simulink model "Can_send_receive"  (R2024a)
settings: Solver=FixedStepAuto  StartTime=0.0  StopTime=20  RelTol=1e-3  EnableMultiTasking=on
undefined symbols (not defined in the file): CAN, FD
libraries: stmutilitieslib x31, simulink x22, stm32blockslib x10, canfdmsglib x6, stm32h7xxblockslib x2
settings Model: STM32="{\"FDCANWrite\":[{\"ID\":\"Can_send_receive:103\"},{\"ID\":\"Can_send_receive:112\"},{\"ID\":\"Can_send_receive:559\"},{\"ID\":\"Can_send_receive:574\"},{\"ID\":\"Can_send_receive:617\"},{\"ID\":\"Can_send_receive:630\"},{\"ID\":\"Can_send_receive:677\"},{\"ID\":\"Can_send_receive:678\"}],\"HardwareInterrupt\":[{\"ID\":\"Can_send_receive:135\"},{\"ID\":\"Can_send_receive:278\"}],\"FDCANRead\":[{\"ID\":\"Can_send_receive:127\"},{\"ID\":\"Can_send_receive:282\"}]}"  Creator=ezeki  LastModifiedBy=ezeki
settings SolverCC: PositivePriorityOrder=on  AutoInsertRateTranBlk=on
settings OptimizationCC: DefaultParameterBehavior=Inlined  EnhancedBackFolding=on  PassReuseOutputArgsAs=Individual arguments  ZeroExternalMemoryAtStartup=off  ZeroInternalMemoryAtStartup=off  MaxStackSize=512  OptimizeBlockOrder=speed  DifferentSizesBufferReuse=on  OptimizationCustomize=off  EfficientTunableParamExpr=on
settings DebuggingCC: ParameterTunabilityLossMsg=error
settings HardwareCC: ProdBitPerPointer=32  ProdBitPerSizeT=32  ProdBitPerPtrDiffT=32  ProdLargestAtomicInteger=Long  ProdLargestAtomicFloat=Double  ProdWordSize=32  ProdLongLongMode=on  ProdHWDeviceType=ARM Compatible->ARM Cortex-M
settings SFSimCC: MATLABDynamicMemAlloc=off
settings RTWCC: Description=Embedded Coder  SystemTargetFile=ert.tlc  HardwareBoard=STM32H7xx Based (Single-core)  TLCOptions="-aInlineSetEventsForThisBaseRateFcn=TLC_FALSE -aSuppressMultiTaskScheduler=TLC_FALSE  -aRateBasedStepFcn=0"  TemplateMakefile=ert_default_tmf  Toolchain=GNU Tools for ARM Embedded Processors  BuildConfiguration=Faster Runs
settings CodeAppCC: ForceParamTrailComments=on  IgnoreCustomStorageClasses=off  OperatorAnnotations=on  SimulinkDataObjDesc=on  SFDataObjDesc=on  InsertBlockDesc=on
settings ERTTargetCC: TargetLangStandard=C99 (ISO)  CodeReplacementLibrary=ARM Cortex-M  ExtModeTransport=3  ExtModeStaticAlloc=on  ExtModeStaticAllocSize=2048  ExtModeMexFile=ext_xcp  ExtModeIntrfLevel=Level2 - Open

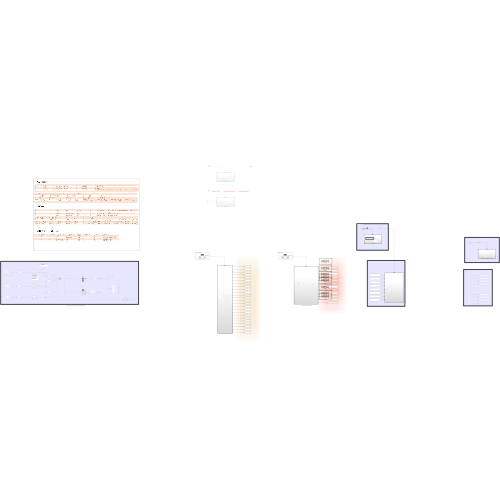
[thumbnail: Simulink's stored preview of the top-level diagram]
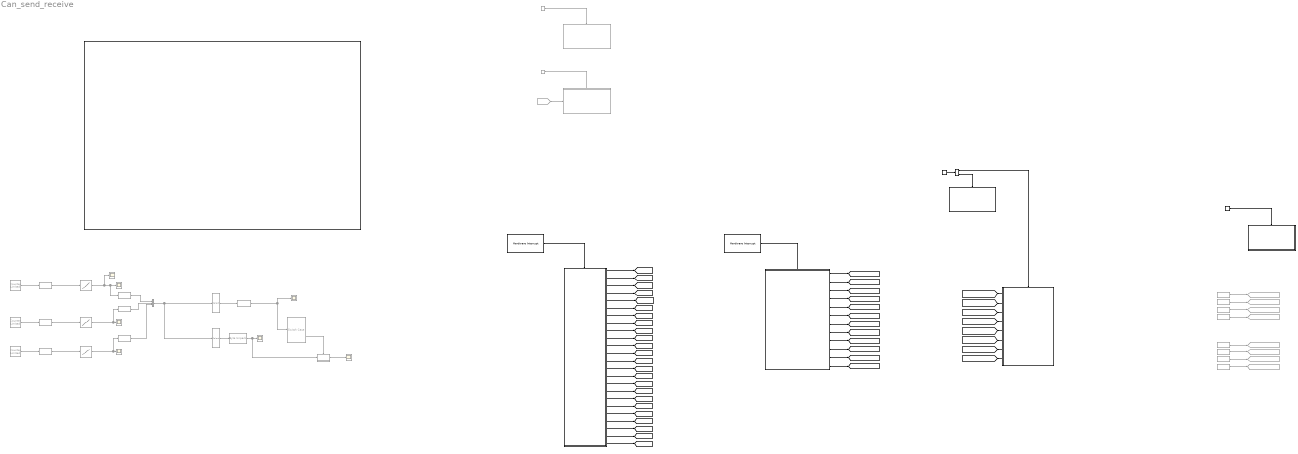
== system Can_send_receive ==
  note: For testing purposes only
  note: CAN 1 information from pedal box and dash.
  note: CAN 2 Receive Data From Inverters
  note: Forwarding Messages From the Inverters to Data Logger
  note: Example On How to send Messages to Inverters
  note: This was made for testing the unmultiplexing of Inverter Messages
  note: Inverter Can Setup
  note: A look up table of CAN ID's which are used to request cyclic transmission of data from the inverters
  note: Counter Selects which ID to send
  note: Byte 0 tells the inverters you are setting up cyclic messaging.
  1-D Lookup Table : Lookup_n-D  Commented=on  NumberOfTableDimensions=1  BreakpointsForDimension1=[0 1 2 3 4 5]  Table=[235 74 168 73 95 138]  InterpMethod=Nearest  InternalRulePriority=Speed  RndMeth=Simplest
  1-D Lookup Table1 : Lookup_n-D  Commented=on  NumberOfTableDimensions=1  BreakpointsForDimension1=[0 1 2 3 4 5]  Table=[25 200 25 200 50 50]  InterpMethod=Nearest  InternalRulePriority=Speed  RndMeth=Simplest
  1-D Lookup Table2 : Lookup_n-D  Commented=on  NumberOfTableDimensions=1  BreakpointsForDimension1=[0 1 2 3 4 5]  Table=[25 200 25 200 50 50]  InterpMethod=Nearest  InternalRulePriority=Speed  RndMeth=Simplest
  10 HZ Send : Subsystem  Commented=on  TreatAsAtomicUnit=on
  10 HZ Send1 : Subsystem  TreatAsAtomicUnit=on
  50 HZ Send Torque Requests to Inverters : Subsystem  TreatAsAtomicUnit=on
  50 HZ Send1 : Subsystem  Commented=on  TreatAsAtomicUnit=on
  Byte Unpack : stmutilitieslib/Byte Unpack  Commented=on  dimensions={[1]}  datatypes={'uint16'}  byteAlign=1  blockPlatform=stm32f4discovery
  Constant{,1..3,5..6,10..11} (8 alike) : Constant  Commented=on  Value=25000
  Counter Limited : simulink/Sources/Counter Limited  Commented=on  uplimit=5  tsamp=0.1
  Counter Limited1 : simulink/Sources/Counter Limited  Commented=on  uplimit=5  tsamp=0.4
  Counter Limited2 : simulink/Sources/Counter Limited  Commented=on  uplimit=5  tsamp=0.7
  Data Type Conversion{1,3,5,16} (4 alike) : DataTypeConversion  Commented=on  OutDataTypeStr=double  SaturateOnIntegerOverflow=off  RndMeth=Floor
  Data Type Conversion2 : DataTypeConversion  Commented=on  OutDataTypeStr=uint8  SaturateOnIntegerOverflow=off  RndMeth=Floor
  Data Type Conversion4 : DataTypeConversion  Commented=on  OutDataTypeStr=uint8  SaturateOnIntegerOverflow=off  RndMeth=Floor
  Data Type Conversion6 : DataTypeConversion  Commented=on  OutDataTypeStr=uint8  SaturateOnIntegerOverflow=off  RndMeth=Floor
  From : From  Commented=on  GotoTag=WSFR
  Function-Call Generator : simulink/Ports & Subsystems/Function-Call Generator  Commented=on  sample_time=0.1  numberOfIterations=1  DisallowWideOutput=off
  Function-Call Generator1 : simulink/Ports & Subsystems/Function-Call Generator  Commented=on  sample_time=0.02  numberOfIterations=1  DisallowWideOutput=off
  Function-Call Generator2 : simulink/Ports & Subsystems/Function-Call Generator  sample_time=0.02  numberOfIterations=1  DisallowWideOutput=off
  Function-Call Generator4 : simulink/Ports & Subsystems/Function-Call Generator  sample_time=0.2  numberOfIterations=1  DisallowWideOutput=off
  Function-Call Split : FunctionCallSplit  IconShape=distinctive  NumOutputPorts=2  OutputPortLayout=default
  Function-Call Subsystem : Subsystem  TreatAsAtomicUnit=on
  Function-Call Subsystem1 : Subsystem  TreatAsAtomicUnit=on
  Goto36 : Goto  Commented=on  GotoTag=CAN_LEFT_Inverter_Bus_Voltage
  Goto37 : Goto  Commented=on  GotoTag=CAN_LEFT_Inverter_Motor_Current
  Goto38 : Goto  Commented=on  GotoTag=CAN_LEFT_Inverter_Motor_Speed
  Goto39 : Goto  Commented=on  GotoTag=CAN_RIGHT_Inverter_Motor_Speed
  Goto41 : Goto  Commented=on  GotoTag=CAN_LEFT_Inverter_Motor_Voltage
  Goto42 : Goto  Commented=on  GotoTag=CAN_RIGHT_Inverter_Bus_Voltage
  Goto45 : Goto  Commented=on  GotoTag=CAN_RIGHT_Inverter_Motor_Current
  Goto47 : Goto  Commented=on  GotoTag=CAN_RIGHT_Inverter_Motor_Voltage
  Hardware Interrupt1 : stm32h7xxblockslib/Hardware Interrupt  ISRGroup=Controller Area Network Flexible Data-Rate (FDCAN)  ISRName=FDCAN2_IT0_IRQHandler  ISRNumber=35  EventsList={ 'off', 'FDCAN2 HPME', '1'; 'off', 'FDCAN2 DRXE', '2'; 'on', 'FDCAN2 RF0NE', '3'; 'off', 'FDCAN2 RF0F', '4'; 'off', 'FDCAN2 RF0L', '5'; 'off', 'FDCAN2 RF0W', '6'; 'off', 'FDCAN2 RF1NE', '7'; 'off', 'FDCAN2 RF1F', '8'; 'off', 'FDCAN2 RF1L', '9'; 'off', 'FDCAN2 RF1W', '10'; 'off', 'FDCAN2 TC', '11'; 'off', 'FDCAN2 TCF', '12'; 'off', 'FDCAN2 TFE', '13'; 'off', 'FDCAN2 TEFN', '14'; 'off', 'FDCAN2 TEFL', '15'; 'off', 'FDCAN2 TEFF', '16'; 'off', 'FDCAN2 TEFW', '17'; 'off', 'FDCAN2 TSW', '18'; 'off', 'FDCAN2 MRAF', '19'; 'off', 'FDCAN2 TOO', '20'; 'off', 'FDCAN2 ELO', '21'; 'off', 'FDCAN2 EP', '22'; 'off', 'FDCAN2 EW', '23'; 'off', 'FDCAN2 BO', '24'; 'off', 'FDCAN2 WDI', '25'; 'off', 'FDCAN2 PEA', '26'; 'off', 'FDCAN2 PED', '27'; 'off', 'FDCAN2 ARA', '28'; 'off', 'Custom event', '29' }  SelectedEvents={'FDCAN2 RF0NE'}  TaskPriority=29  DisablePreemption=off  ClearInterruptFlagsAtEndOfEvent=off  InterruptDefinitionFile=$(TARGET_ROOT)/registry/interrupts/STM32F4xxBased_interrupts.xml  HardwareBoard=STM32H7xx Based  EnableSimPort=off
  Hardware Interrupt3 : stm32h7xxblockslib/Hardware Interrupt  ISRGroup=Controller Area Network Flexible Data-Rate (FDCAN)  ISRName=FDCAN1_IT0_IRQHandler  ISRNumber=34  EventsList={ 'off', 'FDCAN1 HPME', '1'; 'off', 'FDCAN1 DRXE', '2'; 'on', 'FDCAN1 RF0NE', '3'; 'off', 'FDCAN1 RF0F', '4'; 'off', 'FDCAN1 RF0L', '5'; 'off', 'FDCAN1 RF0W', '6'; 'off', 'FDCAN1 RF1NE', '7'; 'off', 'FDCAN1 RF1F', '8'; 'off', 'FDCAN1 RF1L', '9'; 'off', 'FDCAN1 RF1W', '10'; 'off', 'FDCAN1 TC', '11'; 'off', 'FDCAN1 TCF', '12'; 'off', 'FDCAN1 TFE', '13'; 'off', 'FDCAN1 TEFN', '14'; 'off', 'FDCAN1 TEFL', '15'; 'off', 'FDCAN1 TEFF', '16'; 'off', 'FDCAN1 TEFW', '17'; 'off', 'FDCAN1 TSW', '18'; 'off', 'FDCAN1 MRAF', '19'; 'off', 'FDCAN1 TOO', '20'; 'off', 'FDCAN1 ELO', '21'; 'off', 'FDCAN1 EP', '22'; 'off', 'FDCAN1 EW', '23'; 'off', 'FDCAN1 BO', '24'; 'off', 'FDCAN1 WDI', '25'; 'off', 'FDCAN1 PEA', '26'; 'off', 'FDCAN1 PED', '27'; 'off', 'FDCAN1 ARA', '28'; 'off', 'Custom event', '29' }  SelectedEvents={'FDCAN1 RF0NE'}  TaskPriority=30  DisablePreemption=off  ClearInterruptFlagsAtEndOfEvent=off  InterruptDefinitionFile=$(TARGET_ROOT)/registry/interrupts/STM32F4xxBased_interrupts.xml  HardwareBoard=STM32H7xx Based  EnableSimPort=off
  If Action Subsystem1 : Subsystem  Commented=on  TreatAsAtomicUnit=on
  Scope{,1..5,7} (7 alike) : Scope  Commented=on
  Selector : Selector  Commented=on  InputPortWidth=3  IndexOptions=Index vector (dialog)  Indices=[1 ]  OutputSizes=1
  Selector6 : Selector  Commented=on  InputPortWidth=3  IndexOptions=Index vector (dialog)  Indices=[2 3 ]  OutputSizes=1
  Subsystem : Subsystem
      mask Display: image('ALL Can.jpg');
  Switch Case : SwitchCase  Commented=on  CaseConditions={235, 74, 168, 73, 95, 138}
  Triggered Subsystem : Subsystem  TreatAsAtomicUnit=on
  Vector Concatenate : Concatenate  Commented=on  NumInputs=3
  wires:
  Function-Call Generator1/1 -> 50 HZ Send1/Trigger
  Function-Call Generator/1 -> 10 HZ Send/Trigger
  Hardware Interrupt3/1 -> Function-Call Subsystem1/Trigger
  Function-Call Subsystem1/1(Out1) -> [Start_Button]
  Function-Call Subsystem1/2(Out2) -> [SCin]
  Function-Call Subsystem1/3(Out3) -> [SCEstop]
  Function-Call Subsystem1/4(Out4) -> [SCis]
  Function-Call Subsystem1/5(Out5) -> [SCBOTS]
  Function-Call Subsystem1/6(Out6) -> [APPSFail]
  Function-Call Subsystem1/7(Out7) -> [BSEFail]
  Function-Call Subsystem1/8(Out8) -> [SteeringFail]
  Function-Call Subsystem1/9(Out9) -> [APPSMatch]
  Function-Call Subsystem1/10(Out10) -> [BrakesON]
  Function-Call Subsystem1/11(Out11) -> [SoftwareBSPD]
  Function-Call Subsystem1/12(Out12) -> [SoftwareError]
  Function-Call Subsystem1/13(Out13) -> [BSEMatch]
  Function-Call Subsystem1/14(Out14) -> [APPS_Percent]
  Function-Call Subsystem1/15(Out15) -> [Brake_Percent]
  Function-Call Subsystem1/16(Out16) -> [SteeringPercent]
  Function-Call Subsystem1/17(Out17) -> [WSFL]
  Function-Call Subsystem1/18(Out18) -> [WSFR]
  From/1 -> 50 HZ Send1/1(In1)
  Function-Call Subsystem1/19(Out19) -> [BMS_Current]
  Function-Call Subsystem1/20(Out20) -> [BMS_Voltage]
  Function-Call Subsystem1/21(Out21) -> [BMS_SOC]
  Function-Call Subsystem1/22(Out22) -> [BMS_Temprature]
  Function-Call Subsystem1/23(Out23) -> [BMS_Max_CellTemp]
  Function-Call Subsystem1/24(Out24) -> [BMS_Min_CellTemp]
  Hardware Interrupt1/1 -> Function-Call Subsystem/Trigger
  Function-Call Split/2 -> 10 HZ Send1/Trigger
  1-D Lookup Table1/1 -> Data Type Conversion4/1, Scope1/1
  1-D Lookup Table/1 -> Scope2/1, Data Type Conversion2/1, Scope/1
  Counter Limited1/1 -> Data Type Conversion1/1
  Data Type Conversion2/1 -> Vector Concatenate/1
  Counter Limited/1 -> Data Type Conversion16/1
  Data Type Conversion16/1 -> 1-D Lookup Table/1
  Data Type Conversion1/1 -> 1-D Lookup Table1/1
  Data Type Conversion4/1 -> Vector Concatenate/2
  Data Type Conversion3/1 -> Scope4/1, Switch Case/1  "Brakes Percentage"
  Selector/1 -> Data Type Conversion3/1  "Byte 0"
  Vector Concatenate/1 -> Selector6/1, Selector/1
  Data Type Conversion5/1 -> 1-D Lookup Table2/1
  Counter Limited2/1 -> Data Type Conversion5/1
  Data Type Conversion6/1 -> Vector Concatenate/3
  1-D Lookup Table2/1 -> Data Type Conversion6/1, Scope3/1
  Switch Case/6 -> If Action Subsystem1/Action
  If Action Subsystem1/1(Out1) -> Scope5/1
  Selector6/1 -> Byte Unpack/1  "Byte 0"
  Byte Unpack/1 -> If Action Subsystem1/1(In1), Scope7/1
  Function-Call Subsystem/2(Out2) -> [CAN_LEFT_Inverter_IGBT_temp]
  Function-Call Subsystem/1(Out1) -> [CAN_LEFT_Inverter_Bus_Voltage]
  Function-Call Subsystem/3(Out3) -> [CAN_LEFT_Inverter_Motor_Speed]
  Function-Call Subsystem/4(Out4) -> [CAN_LEFT_Inverter_Motor_Temp]
  Function-Call Subsystem/5(Out5) -> [CAN_LEFT_Inverter_Motor_Current]
  Function-Call Subsystem/6(Out6) -> [CAN_LEFT_Inverter_Motor_Voltage]
  Function-Call Subsystem/7(Out7) -> [CAN_RIGHT_Inverter_Bus_Voltage]
  Function-Call Subsystem/8(Out8) -> [CAN_RIGHT_Inverter_IGBT_temp]
  Function-Call Subsystem/9(Out9) -> [CAN_RIGHT_Inverter_Motor_Speed]
  Function-Call Subsystem/10(Out10) -> [CAN_RIGHT_Inverter_Motor_Temp]
  Function-Call Subsystem/11(Out11) -> [CAN_RIGHT_Inverter_Motor_Current]
  Function-Call Subsystem/12(Out12) -> [CAN_RIGHT_Inverter_Motor_Voltage]
  Function-Call Generator2/1 -> 50 HZ Send Torque Requests to Inverters/Trigger  "50Hz"
  [CAN_LEFT_Inverter_Bus_Voltage] -> Triggered Subsystem/1(In1)
  [CAN_LEFT_Inverter_Motor_Speed] -> Triggered Subsystem/2(In2)
  [CAN_LEFT_Inverter_Motor_Current] -> Triggered Subsystem/3(In3)
  [CAN_LEFT_Inverter_Motor_Voltage] -> Triggered Subsystem/4(In4)
  [CAN_RIGHT_Inverter_Bus_Voltage] -> Triggered Subsystem/5(In5)
  [CAN_RIGHT_Inverter_Motor_Speed] -> Triggered Subsystem/6(In6)
  [CAN_RIGHT_Inverter_Motor_Current] -> Triggered Subsystem/7(In7)
  [CAN_RIGHT_Inverter_Motor_Voltage] -> Triggered Subsystem/8(In8)
  Constant/1 -> Goto36/1
  Constant2/1 -> Goto38/1
  Constant5/1 -> Goto41/1
  Constant6/1 -> Goto42/1
  Constant10/1 -> Goto45/1
  Constant11/1 -> Goto47/1
  Constant1/1 -> Goto37/1
  Constant3/1 -> Goto39/1
  ? -> ?
  ? -> ?
  ? -> ?
  ? -> ?
  Function-Call Split/1 -> Triggered Subsystem/Trigger  "10Hz"
  Function-Call Generator4/1 -> Function-Call Split/1  "10Hz"

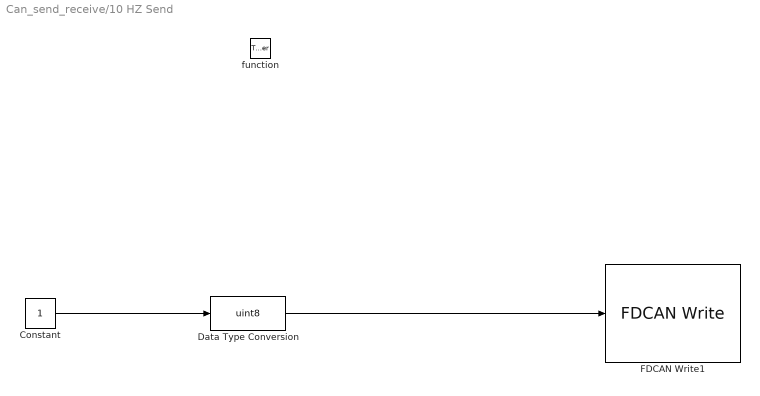
== system Can_send_receive/10 HZ Send ==
  function : TriggerPort  TriggerType=function-call  VariantControl=(inherit)
  Constant : Constant
  Data Type Conversion : DataTypeConversion  OutDataTypeStr=uint8  SaturateOnIntegerOverflow=off  RndMeth=Floor
  FDCAN Write1 : stm32blockslib/FDCAN Write  FDCANModule=FDCAN1  BlockMode=Transmit  OperationReadMode=Data  OperationWriteMode=Data  ReadSource=FIFO 0  BufferNumber=0  OutputTypeReadMode=Unpacked  DataFormatWriteMode=Raw data  CANFrameType=CAN  IdentifierTypeVia=Dialog  IdentifierType=Standard (11-bit identifier)  IdentifierVia=Dialog  Identifier=1200  DataLengthVia=Dialog  DataLength=1  OutputIdType=off  IsBitRateSwitchingEnabled=off  TransmitRemoteFrame=off  OutputFrameType=off  OutputBRS=off  OutputRemoteFrame=off  OutputTxFifoLevel=off  OutputRxFifoLevel=off  OutputStatus=off  Timeout=2  SampleTime=-1
      settings: LibrarySourceBlock=stm32l5xxblockslib/FDCAN Write
  wires:
  Constant/1 -> Data Type Conversion/1
  Data Type Conversion/1 -> FDCAN Write1/1

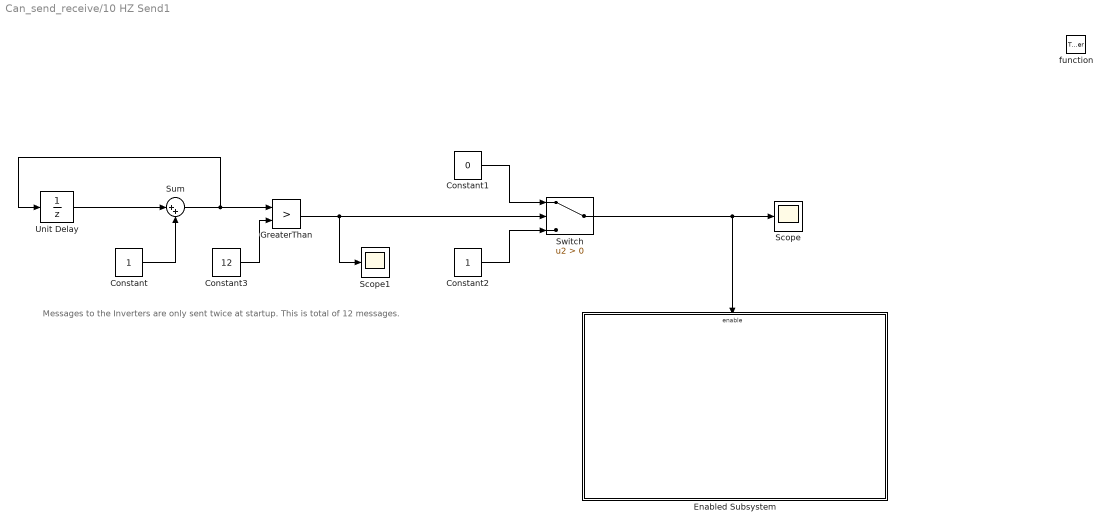
== system Can_send_receive/10 HZ Send1 ==
  note: Messages to the Inverters are only sent twice at startup. This is total of 12 messages.
  function : TriggerPort  TriggerType=function-call  VariantControl=(inherit)
  Constant : Constant
  Constant1 : Constant  Value=0
  Constant2 : Constant
  Constant3 : Constant  Value=12
  Enabled Subsystem : Subsystem  TreatAsAtomicUnit=on
  GreaterThan : RelationalOperator  Operator=>  OutDataTypeStr=boolean  RndMeth=Simplest  InputSameDT=off
  Scope : Scope
  Scope1 : Scope
  Sum : Sum  Inputs=|++
  Switch : Switch  Criteria=u2 > Threshold  SaturateOnIntegerOverflow=off  InputSameDT=off
  Unit Delay : UnitDelay  SampleTime=-1  HasFrameUpgradeWarning=on
  wires:
  Constant/1 -> Sum/2
  Unit Delay/1 -> Sum/1
  Sum/1 -> GreaterThan/1, Unit Delay/1
  Constant1/1 -> Switch/1
  Constant2/1 -> Switch/3
  Constant3/1 -> GreaterThan/2
  GreaterThan/1 -> Scope1/1, Switch/2
  Switch/1 -> Enabled Subsystem/Enable, Scope/1

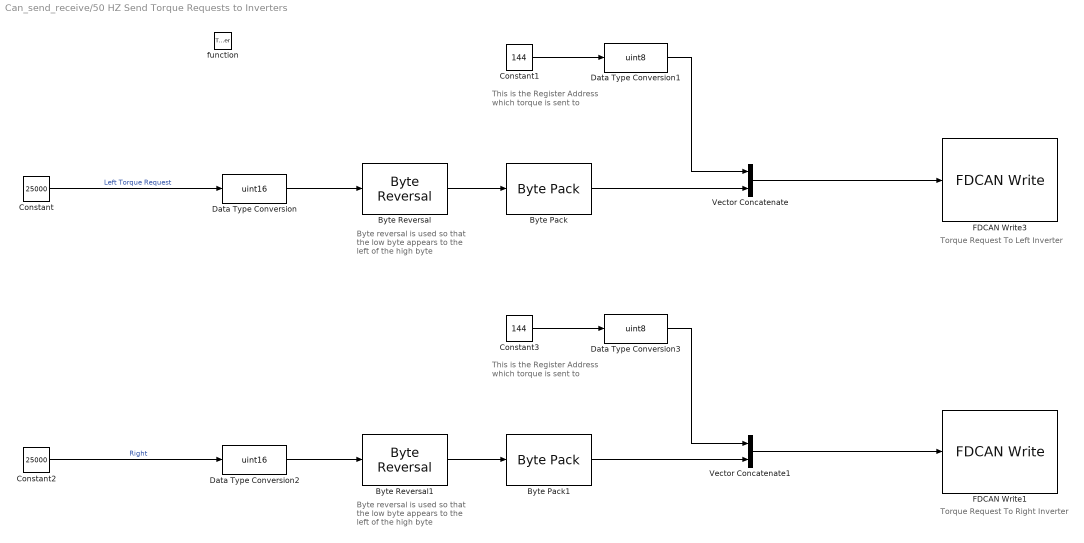
== system Can_send_receive/50 HZ Send Torque Requests to Inverters ==
  note: This is the Register Address which torque is sent to
  note: Torque Request To Left Inverter
  note: Byte reversal is used so that the low byte appears to the left of the high byte
  note: This is the Register Address which torque is sent to
  note: Byte reversal is used so that the low byte appears to the left of the high byte
  note: Torque Request To Right Inverter
  function : TriggerPort  TriggerType=function-call  VariantControl=(inherit)
  Byte Pack : stmutilitieslib/Byte Pack  datatypes={'uint16'}  byteAlign=1  blockPlatform=stm32f4discovery
  Byte Pack1 : stmutilitieslib/Byte Pack  datatypes={'uint16'}  byteAlign=1  blockPlatform=stm32f4discovery
  Byte Reversal : stmutilitieslib/Byte Reversal  numInp=1  blockPlatform=stm32f4discovery
  Byte Reversal1 : stmutilitieslib/Byte Reversal  numInp=1  blockPlatform=stm32f4discovery
  Constant : Constant  Value=25000
  Constant1 : Constant  Value=144
  Constant2 : Constant  Value=25000
  Constant3 : Constant  Value=144
  Data Type Conversion : DataTypeConversion  OutDataTypeStr=uint16  SaturateOnIntegerOverflow=off  RndMeth=Floor
  Data Type Conversion1 : DataTypeConversion  OutDataTypeStr=uint8  SaturateOnIntegerOverflow=off  RndMeth=Floor
  Data Type Conversion2 : DataTypeConversion  OutDataTypeStr=uint16  SaturateOnIntegerOverflow=off  RndMeth=Floor
  Data Type Conversion3 : DataTypeConversion  OutDataTypeStr=uint8  SaturateOnIntegerOverflow=off  RndMeth=Floor
  FDCAN Write1 : stm32blockslib/FDCAN Write  FDCANModule=FDCAN2  BlockMode=Transmit  OperationReadMode=Data  OperationWriteMode=Data  ReadSource=FIFO 0  BufferNumber=0  OutputTypeReadMode=Unpacked  DataFormatWriteMode=Raw data  CANFrameType=CAN  IdentifierTypeVia=Dialog  IdentifierType=Standard (11-bit identifier)  IdentifierVia=Dialog  Identifier=529  DataLengthVia=Dialog  DataLength=3  OutputIdType=off  IsBitRateSwitchingEnabled=off  TransmitRemoteFrame=off  OutputFrameType=off  OutputBRS=off  OutputRemoteFrame=off  OutputTxFifoLevel=off  OutputRxFifoLevel=off  OutputStatus=off  Timeout=1  SampleTime=-1
      settings: LibrarySourceBlock=stm32l5xxblockslib/FDCAN Write
  FDCAN Write3 : stm32blockslib/FDCAN Write  FDCANModule=FDCAN2  BlockMode=Transmit  OperationReadMode=Data  OperationWriteMode=Data  ReadSource=FIFO 0  BufferNumber=0  OutputTypeReadMode=Unpacked  DataFormatWriteMode=Raw data  CANFrameType=CAN  IdentifierTypeVia=Dialog  IdentifierType=Standard (11-bit identifier)  IdentifierVia=Dialog  Identifier=528  DataLengthVia=Dialog  DataLength=3  OutputIdType=off  IsBitRateSwitchingEnabled=off  TransmitRemoteFrame=off  OutputFrameType=off  OutputBRS=off  OutputRemoteFrame=off  OutputTxFifoLevel=off  OutputRxFifoLevel=off  OutputStatus=off  Timeout=1  SampleTime=-1
      settings: LibrarySourceBlock=stm32l5xxblockslib/FDCAN Write
  Vector Concatenate : Concatenate
  Vector Concatenate1 : Concatenate
  wires:
  Constant/1 -> Data Type Conversion/1  "Left Torque Request"
  Data Type Conversion/1 -> Byte Reversal/1
  Byte Pack/1 -> Vector Concatenate/2
  Byte Reversal/1 -> Byte Pack/1
  Vector Concatenate/1 -> FDCAN Write3/1
  Constant1/1 -> Data Type Conversion1/1
  Data Type Conversion1/1 -> Vector Concatenate/1
  Data Type Conversion2/1 -> Byte Reversal1/1
  Vector Concatenate1/1 -> FDCAN Write1/1
  Byte Pack1/1 -> Vector Concatenate1/2
  Constant2/1 -> Data Type Conversion2/1  "Right"
  Data Type Conversion3/1 -> Vector Concatenate1/1
  Byte Reversal1/1 -> Byte Pack1/1
  Constant3/1 -> Data Type Conversion3/1

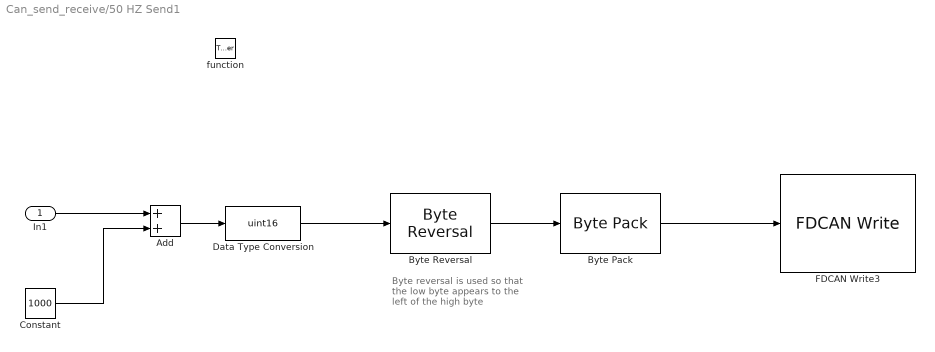
== system Can_send_receive/50 HZ Send1 ==
  note: Byte reversal is used so that the low byte appears to the left of the high byte
  In1 : Inport
  function : TriggerPort  TriggerType=function-call  VariantControl=(inherit)
  Add : Sum
  Byte Pack : stmutilitieslib/Byte Pack  datatypes={'uint16'}  byteAlign=1  blockPlatform=stm32f4discovery
  Byte Reversal : stmutilitieslib/Byte Reversal  numInp=1  blockPlatform=stm32f4discovery
  Constant : Constant  Value=1000
  Data Type Conversion : DataTypeConversion  OutDataTypeStr=uint16  SaturateOnIntegerOverflow=off  RndMeth=Floor
  FDCAN Write3 : stm32blockslib/FDCAN Write  FDCANModule=FDCAN1  BlockMode=Transmit  OperationReadMode=Data  OperationWriteMode=Data  ReadSource=FIFO 0  BufferNumber=0  OutputTypeReadMode=Unpacked  DataFormatWriteMode=Raw data  CANFrameType=CAN  IdentifierTypeVia=Dialog  IdentifierType=Standard (11-bit identifier)  IdentifierVia=Dialog  Identifier=1000  DataLengthVia=Dialog  DataLength=2  OutputIdType=off  IsBitRateSwitchingEnabled=off  TransmitRemoteFrame=off  OutputFrameType=off  OutputBRS=off  OutputRemoteFrame=off  OutputTxFifoLevel=off  OutputRxFifoLevel=off  OutputStatus=off  Timeout=1  SampleTime=-1
      settings: LibrarySourceBlock=stm32l5xxblockslib/FDCAN Write
  wires:
  Add/1 -> Data Type Conversion/1
  In1/1 -> Add/1
  Constant/1 -> Add/2
  Data Type Conversion/1 -> Byte Reversal/1
  Byte Pack/1 -> FDCAN Write3/1
  Byte Reversal/1 -> Byte Pack/1

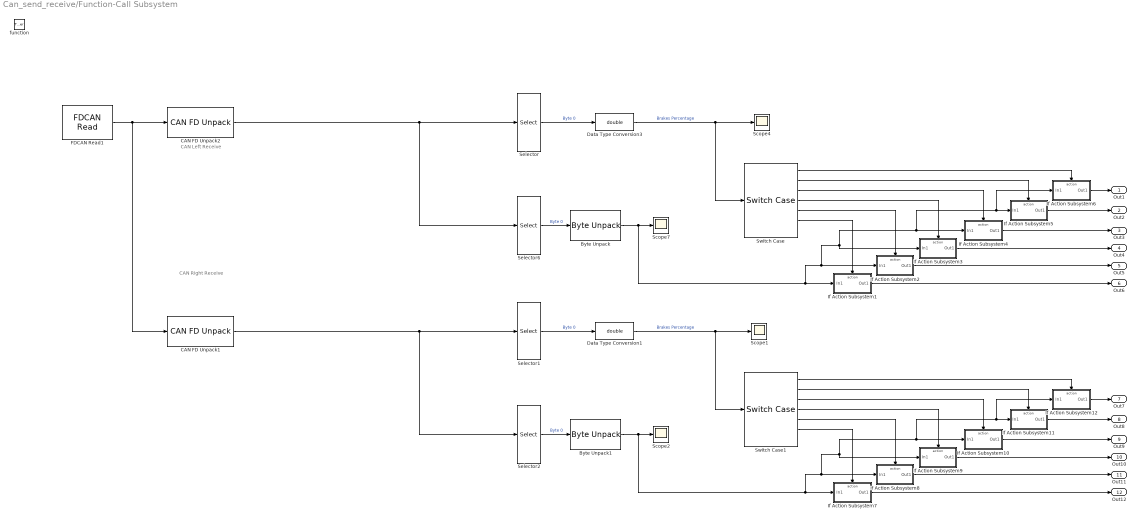
== system Can_send_receive/Function-Call Subsystem ==
  note: CAN Left Receive
  note: CAN Right Receive
  function : TriggerPort  TriggerType=function-call  VariantControl=(inherit)
  Byte Unpack : stmutilitieslib/Byte Unpack  dimensions={[1]}  datatypes={'uint16'}  byteAlign=1  blockPlatform=stm32f4discovery
  Byte Unpack1 : stmutilitieslib/Byte Unpack  dimensions={[1]}  datatypes={'uint16'}  byteAlign=1  blockPlatform=stm32f4discovery
  CAN FD Unpack1 : canfdmsglib/CAN FD Unpack  MsgList=(none)  MsgName=Msg  ProtocolMode=CAN  MsgIDType=Standard (11-bit identifier)  MsgIdentifier=401  MsgLength=3  SignalInfo={}  IDPort=off  TimestampPort=off  ErrorPort=off  RemotePort=off  LengthPort=off  StatusPort=off  BRSPort=off  ESIPort=off  DLCPort=off  ApplyMinMax=off
      settings: LibrarySourceBlock=stmutilitieslib/CAN FD Unpack  DataFormat=raw data
  CAN FD Unpack2 : canfdmsglib/CAN FD Unpack  MsgList=(none)  MsgName=Msg  ProtocolMode=CAN  MsgIDType=Standard (11-bit identifier)  MsgIdentifier=400  MsgLength=3  SignalInfo={}  IDPort=off  TimestampPort=off  ErrorPort=off  RemotePort=off  LengthPort=off  StatusPort=off  BRSPort=off  ESIPort=off  DLCPort=off  ApplyMinMax=off
      settings: LibrarySourceBlock=stmutilitieslib/CAN FD Unpack  DataFormat=raw data
  Data Type Conversion1 : DataTypeConversion  OutDataTypeStr=double  SaturateOnIntegerOverflow=off  RndMeth=Floor
  Data Type Conversion3 : DataTypeConversion  OutDataTypeStr=double  SaturateOnIntegerOverflow=off  RndMeth=Floor
  FDCAN Read1 : stm32blockslib/FDCAN Read  FDCANModule=FDCAN2  BlockMode=Receive  OperationReadMode=Data  OperationWriteMode=Data  ReadSource=FIFO 0  BufferNumber=0  OutputTypeReadMode=Packed  DataFormatWriteMode=Raw data  CANFrameType=CAN-FD  IdentifierTypeVia=Dialog  IdentifierType=Standard (11-bit identifier)  IdentifierVia=Inport  Identifier=100  DataLengthVia=Inport  DataLength=64  OutputIdType=off  IsBitRateSwitchingEnabled=off  TransmitRemoteFrame=off  OutputFrameType=off  OutputBRS=off  OutputRemoteFrame=off  OutputTxFifoLevel=off  OutputRxFifoLevel=off  OutputStatus=off  Timeout=0.001  SampleTime=-1
      settings: LibrarySourceBlock=stm32l5xxblockslib/FDCAN Read
  If Action Subsystem1 : Subsystem  TreatAsAtomicUnit=on
  If Action Subsystem10 : Subsystem  TreatAsAtomicUnit=on
  If Action Subsystem11 : Subsystem  TreatAsAtomicUnit=on
  If Action Subsystem12 : Subsystem  TreatAsAtomicUnit=on
  If Action Subsystem2 : Subsystem  TreatAsAtomicUnit=on
  If Action Subsystem3 : Subsystem  TreatAsAtomicUnit=on
  If Action Subsystem4 : Subsystem  TreatAsAtomicUnit=on
  If Action Subsystem5 : Subsystem  TreatAsAtomicUnit=on
  If Action Subsystem6 : Subsystem  TreatAsAtomicUnit=on
  If Action Subsystem7 : Subsystem  TreatAsAtomicUnit=on
  If Action Subsystem8 : Subsystem  TreatAsAtomicUnit=on
  If Action Subsystem9 : Subsystem  TreatAsAtomicUnit=on
  Scope{1..2,4,7} (4 alike) : Scope
  Selector : Selector  InputPortWidth=3  IndexOptions=Index vector (dialog)  Indices=[1 ]  OutputSizes=1
  Selector1 : Selector  InputPortWidth=3  IndexOptions=Index vector (dialog)  Indices=[1 ]  OutputSizes=1
  Selector2 : Selector  InputPortWidth=3  IndexOptions=Index vector (dialog)  Indices=[2 3 ]  OutputSizes=1
  Selector6 : Selector  InputPortWidth=3  IndexOptions=Index vector (dialog)  Indices=[2 3 ]  OutputSizes=1
  Switch Case : SwitchCase  CaseConditions={235, 74, 168, 73, 95, 138}
  Switch Case1 : SwitchCase  CaseConditions={235, 74, 168, 73, 95, 138}
  Out1 : Outport
  Out2 : Outport  Port=2
  Out3 : Outport  Port=3
  Out4 : Outport  Port=4
  Out5 : Outport  Port=5
  Out6 : Outport  Port=6
  Out7 : Outport  Port=7
  Out8 : Outport  Port=8
  Out9 : Outport  Port=9
  Out10 : Outport  Port=10
  Out11 : Outport  Port=11
  Out12 : Outport  Port=12
  wires:
  FDCAN Read1/1 -> CAN FD Unpack1/1, CAN FD Unpack2/1
  CAN FD Unpack2/1 -> Selector6/1, Selector/1
  Selector/1 -> Data Type Conversion3/1  "Byte 0"
  Data Type Conversion3/1 -> Scope4/1, Switch Case/1  "Brakes Percentage"
  Byte Unpack/1 -> If Action Subsystem6/1(In1), If Action Subsystem5/1(In1), If Action Subsystem4/1(In1), If Action Subsystem3/1(In1), If Action Subsystem2/1(In1), If Action Subsystem1/1(In1), Scope7/1
  Selector6/1 -> Byte Unpack/1  "Byte 0"
  Switch Case/6 -> If Action Subsystem1/Action
  If Action Subsystem1/1(Out1) -> Out6/1
  Switch Case/5 -> If Action Subsystem2/Action
  Switch Case/4 -> If Action Subsystem3/Action
  Switch Case/3 -> If Action Subsystem4/Action
  Switch Case/2 -> If Action Subsystem5/Action
  Switch Case/1 -> If Action Subsystem6/Action
  If Action Subsystem6/1(Out1) -> Out1/1
  If Action Subsystem5/1(Out1) -> Out2/1
  If Action Subsystem4/1(Out1) -> Out3/1
  If Action Subsystem2/1(Out1) -> Out5/1
  If Action Subsystem3/1(Out1) -> Out4/1
  Selector2/1 -> Byte Unpack1/1  "Byte 0"
  Switch Case1/6 -> If Action Subsystem7/Action
  Byte Unpack1/1 -> If Action Subsystem12/1(In1), If Action Subsystem11/1(In1), If Action Subsystem10/1(In1), If Action Subsystem9/1(In1), If Action Subsystem8/1(In1), If Action Subsystem7/1(In1), Scope2/1
  Data Type Conversion1/1 -> Scope1/1, Switch Case1/1  "Brakes Percentage"
  If Action Subsystem10/1(Out1) -> Out9/1
  Switch Case1/2 -> If Action Subsystem11/Action
  Switch Case1/3 -> If Action Subsystem10/Action
  If Action Subsystem7/1(Out1) -> Out12/1
  Selector1/1 -> Data Type Conversion1/1  "Byte 0"
  If Action Subsystem11/1(Out1) -> Out8/1
  If Action Subsystem9/1(Out1) -> Out10/1
  If Action Subsystem12/1(Out1) -> Out7/1
  Switch Case1/5 -> If Action Subsystem8/Action
  Switch Case1/4 -> If Action Subsystem9/Action
  If Action Subsystem8/1(Out1) -> Out11/1
  Switch Case1/1 -> If Action Subsystem12/Action
  CAN FD Unpack1/1 -> Selector2/1, Selector1/1

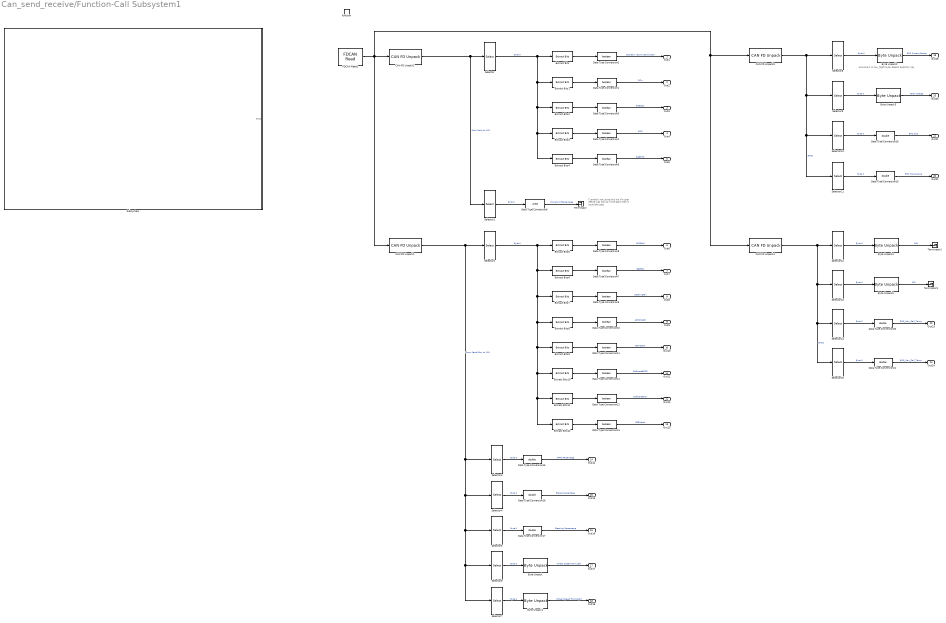
== system Can_send_receive/Function-Call Subsystem1 ==
  note: Assume it is low_hight byte, doesnt explicity say
  note: Currently not using this but if a user define was set up in the dash then it could be used.
  function : TriggerPort  TriggerType=function-call  VariantControl=(inherit)
  Byte Unpack{,1..5} (6 alike) : stmutilitieslib/Byte Unpack  dimensions={[1]}  datatypes={'uint16'}  byteAlign=1  blockPlatform=stm32f4discovery
  CAN FD Unpack1 : canfdmsglib/CAN FD Unpack  MsgList=(none)  MsgName=Msg  ProtocolMode=CAN  MsgIDType=Standard (11-bit identifier)  MsgIdentifier=1  MsgLength=8  SignalInfo={}  IDPort=off  TimestampPort=off  ErrorPort=off  RemotePort=off  LengthPort=off  StatusPort=off  BRSPort=off  ESIPort=off  DLCPort=off  ApplyMinMax=off
      settings: LibrarySourceBlock=stmutilitieslib/CAN FD Unpack  DataFormat=raw data
  CAN FD Unpack2 : canfdmsglib/CAN FD Unpack  MsgList=(none)  MsgName=Msg  ProtocolMode=CAN  MsgIDType=Standard (11-bit identifier)  MsgIdentifier=2  MsgLength=8  SignalInfo={}  IDPort=off  TimestampPort=off  ErrorPort=off  RemotePort=off  LengthPort=off  StatusPort=off  BRSPort=off  ESIPort=off  DLCPort=off  ApplyMinMax=off
      settings: LibrarySourceBlock=stmutilitieslib/CAN FD Unpack  DataFormat=raw data
  CAN FD Unpack3 : canfdmsglib/CAN FD Unpack  MsgList=(none)  MsgName=Msg  ProtocolMode=CAN  MsgIDType=Standard (11-bit identifier)  MsgIdentifier=4  MsgLength=8  SignalInfo={}  IDPort=off  TimestampPort=off  ErrorPort=off  RemotePort=off  LengthPort=off  StatusPort=off  BRSPort=off  ESIPort=off  DLCPort=off  ApplyMinMax=off
      settings: LibrarySourceBlock=stmutilitieslib/CAN FD Unpack  DataFormat=raw data
  CAN FD Unpack4 : canfdmsglib/CAN FD Unpack  MsgList=(none)  MsgName=Msg  ProtocolMode=CAN  MsgIDType=Standard (11-bit identifier)  MsgIdentifier=5  MsgLength=8  SignalInfo={}  IDPort=off  TimestampPort=off  ErrorPort=off  RemotePort=off  LengthPort=off  StatusPort=off  BRSPort=off  ESIPort=off  DLCPort=off  ApplyMinMax=off
      settings: LibrarySourceBlock=stmutilitieslib/CAN FD Unpack  DataFormat=raw data
  Data Type Conversion{1..5,7..14} (13 alike) : DataTypeConversion  OutDataTypeStr=boolean  SaturateOnIntegerOverflow=off  RndMeth=Floor
  Data Type Conversion{15..21} (7 alike) : DataTypeConversion  OutDataTypeStr=double  SaturateOnIntegerOverflow=off  RndMeth=Floor
  Data Type Conversion6 : DataTypeConversion  OutDataTypeStr=uint8  SaturateOnIntegerOverflow=off  RndMeth=Floor
  Extract Bits : simulink/Logic and Bit Operations/Extract Bits  bitsToExtract=Range of bits  numBits=8  bitIdxRange=[0]  outScalingMode=Treat bit field as an integer
  Extract Bits1 : simulink/Logic and Bit Operations/Extract Bits  bitsToExtract=Range of bits  numBits=8  bitIdxRange=[3]  outScalingMode=Treat bit field as an integer
  Extract Bits10 : simulink/Logic and Bit Operations/Extract Bits  bitsToExtract=Range of bits  numBits=8  bitIdxRange=[5]  outScalingMode=Treat bit field as an integer
  Extract Bits11 : simulink/Logic and Bit Operations/Extract Bits  bitsToExtract=Range of bits  numBits=8  bitIdxRange=[6]  outScalingMode=Treat bit field as an integer
  Extract Bits12 : simulink/Logic and Bit Operations/Extract Bits  bitsToExtract=Range of bits  numBits=8  bitIdxRange=[7]  outScalingMode=Treat bit field as an integer
  Extract Bits2 : simulink/Logic and Bit Operations/Extract Bits  bitsToExtract=Range of bits  numBits=8  bitIdxRange=[4]  outScalingMode=Treat bit field as an integer
  Extract Bits3 : simulink/Logic and Bit Operations/Extract Bits  bitsToExtract=Range of bits  numBits=8  bitIdxRange=[5]  outScalingMode=Treat bit field as an integer
  Extract Bits4 : simulink/Logic and Bit Operations/Extract Bits  bitsToExtract=Range of bits  numBits=8  bitIdxRange=[6]  outScalingMode=Treat bit field as an integer
  Extract Bits5 : simulink/Logic and Bit Operations/Extract Bits  bitsToExtract=Range of bits  numBits=8  bitIdxRange=[0]  outScalingMode=Treat bit field as an integer
  Extract Bits6 : simulink/Logic and Bit Operations/Extract Bits  bitsToExtract=Range of bits  numBits=8  bitIdxRange=[1]  outScalingMode=Treat bit field as an integer
  Extract Bits7 : simulink/Logic and Bit Operations/Extract Bits  bitsToExtract=Range of bits  numBits=8  bitIdxRange=[2]  outScalingMode=Treat bit field as an integer
  Extract Bits8 : simulink/Logic and Bit Operations/Extract Bits  bitsToExtract=Range of bits  numBits=8  bitIdxRange=[3]  outScalingMode=Treat bit field as an integer
  Extract Bits9 : simulink/Logic and Bit Operations/Extract Bits  bitsToExtract=Range of bits  numBits=8  bitIdxRange=[4]  outScalingMode=Treat bit field as an integer
  FDCAN Read1 : stm32blockslib/FDCAN Read  FDCANModule=FDCAN1  BlockMode=Receive  OperationReadMode=Data  OperationWriteMode=Data  ReadSource=FIFO 0  BufferNumber=0  OutputTypeReadMode=Packed  DataFormatWriteMode=Raw data  CANFrameType=CAN-FD  IdentifierTypeVia=Dialog  IdentifierType=Standard (11-bit identifier)  IdentifierVia=Inport  Identifier=100  DataLengthVia=Inport  DataLength=64  OutputIdType=off  IsBitRateSwitchingEnabled=off  TransmitRemoteFrame=off  OutputFrameType=off  OutputBRS=off  OutputRemoteFrame=off  OutputTxFifoLevel=off  OutputRxFifoLevel=off  OutputStatus=off  Timeout=0.001  SampleTime=-1
      settings: LibrarySourceBlock=stm32l5xxblockslib/FDCAN Read
  Selector : Selector  InputPortWidth=8  IndexOptions=Index vector (dialog)  Indices=[1 ]  OutputSizes=1
  Selector1 : Selector  InputPortWidth=8  IndexOptions=Index vector (dialog)  Indices=[2 ]  OutputSizes=1
  Selector{10..11,14..15} (4 alike) : Selector  InputPortWidth=8  IndexOptions=Index vector (dialog)  Indices=[5 ]  OutputSizes=1
  Selector12 : Selector  InputPortWidth=8  IndexOptions=Index vector (dialog)  Indices=[1 2 ]  OutputSizes=1
  Selector13 : Selector  InputPortWidth=8  IndexOptions=Index vector (dialog)  Indices=[3 4 ]  OutputSizes=1
  Selector2 : Selector  InputPortWidth=8  IndexOptions=Index vector (dialog)  Indices=[1 ]  OutputSizes=1
  Selector3 : Selector  InputPortWidth=8  IndexOptions=Index vector (dialog)  Indices=[2 ]  OutputSizes=1
  Selector4 : Selector  InputPortWidth=8  IndexOptions=Index vector (dialog)  Indices=[3 ]  OutputSizes=1
  Selector5 : Selector  InputPortWidth=8  IndexOptions=Index vector (dialog)  Indices=[4 ]  OutputSizes=1
  Selector6 : Selector  InputPortWidth=8  IndexOptions=Index vector (dialog)  Indices=[5 6 ]  OutputSizes=1
  Selector7 : Selector  InputPortWidth=8  IndexOptions=Index vector (dialog)  Indices=[7 8 ]  OutputSizes=1
  Selector8 : Selector  InputPortWidth=8  IndexOptions=Index vector (dialog)  Indices=[1 2 ]  OutputSizes=1
  Selector9 : Selector  InputPortWidth=8  IndexOptions=Index vector (dialog)  Indices=[3 4 ]  OutputSizes=1
  Subsystem : Subsystem
      mask Display: image('ALL Can.jpg');
  Terminator : Terminator
  Terminator1 : Terminator
  Terminator2 : Terminator
  Out1 : Outport
  Out2 : Outport  Port=2
  Out3 : Outport  Port=3
  Out4 : Outport  Port=4
  Out5 : Outport  Port=5
  Out6 : Outport  Port=6
  Out7 : Outport  Port=7
  Out8 : Outport  Port=8
  Out9 : Outport  Port=9
  Out10 : Outport  Port=10
  Out11 : Outport  Port=11
  Out12 : Outport  Port=12
  Out13 : Outport  Port=13
  Out14 : Outport  Port=14
  Out15 : Outport  Port=15
  Out16 : Outport  Port=16
  Out17 : Outport  Port=17
  Out18 : Outport  Port=18
  Out19 : Outport  Port=19
  Out20 : Outport  Port=20
  Out21 : Outport  Port=21
  Out22 : Outport  Port=22
  Out23 : Outport  Port=23
  Out24 : Outport  Port=24
  wires:
  CAN FD Unpack2/1 -> Selector1/1, Selector/1  "From Dash to VCU"
  FDCAN Read1/1 -> CAN FD Unpack1/1, CAN FD Unpack4/1, CAN FD Unpack3/1, CAN FD Unpack2/1
  Selector/1 -> Extract Bits4/1, Extract Bits3/1, Extract Bits2/1, Extract Bits1/1, Extract Bits/1  "Byte 0"
  Extract Bits/1 -> Data Type Conversion2/1
  Data Type Conversion2/1 -> Out1/1  "Boolean yes/no start button"
  Extract Bits1/1 -> Data Type Conversion1/1
  Data Type Conversion1/1 -> Out2/1  "SCin"
  Extract Bits2/1 -> Data Type Conversion3/1
  Data Type Conversion3/1 -> Out3/1  "SCEstop"
  Extract Bits3/1 -> Data Type Conversion4/1
  Data Type Conversion4/1 -> Out4/1  "SCIS"
  Extract Bits4/1 -> Data Type Conversion5/1
  Data Type Conversion5/1 -> Out5/1  "SCBOTS"
  Selector1/1 -> Data Type Conversion6/1  "Byte 0"
  Data Type Conversion6/1 -> Terminator/1  "PowerLimitPercentage"
  CAN FD Unpack1/1 -> Selector7/1, Selector6/1, Selector5/1, Selector4/1, Selector3/1, Selector2/1  "From Pedal Box to VCU"
  Data Type Conversion9/1 -> Out8/1  "SteeringFail"
  Extract Bits7/1 -> Data Type Conversion9/1
  Extract Bits6/1 -> Data Type Conversion7/1
  Extract Bits9/1 -> Data Type Conversion11/1
  Extract Bits5/1 -> Data Type Conversion8/1
  Extract Bits8/1 -> Data Type Conversion10/1
  Data Type Conversion7/1 -> Out7/1  "BSEFail"
  Data Type Conversion8/1 -> Out6/1  "APPSFail"
  Data Type Conversion10/1 -> Out9/1  "APPSMatch"
  Data Type Conversion11/1 -> Out10/1  "BrakesON"
  Extract Bits11/1 -> Data Type Conversion12/1
  Extract Bits12/1 -> Data Type Conversion13/1
  Data Type Conversion13/1 -> Out13/1  "BSEMatch"
  Selector2/1 -> Extract Bits12/1, Extract Bits11/1, Extract Bits10/1, Extract Bits9/1, Extract Bits8/1, Extract Bits7/1, Extract Bits6/1, Extract Bits5/1  "Byte 0"
  Data Type Conversion12/1 -> Out12/1  "SoftwareError"
  Data Type Conversion14/1 -> Out11/1  "SoftwareBSPD"
  Extract Bits10/1 -> Data Type Conversion14/1
  Selector3/1 -> Data Type Conversion15/1  "Byte 0"
  Data Type Conversion15/1 -> Out14/1  "APPS Percentage"
  Selector4/1 -> Data Type Conversion16/1  "Byte 0"
  Data Type Conversion16/1 -> Out15/1  "Brakes Percentage"
  Selector5/1 -> Data Type Conversion17/1  "Byte 0"
  Data Type Conversion17/1 -> Out16/1  "Steering Percentage"
  Selector6/1 -> Byte Unpack/1  "Byte 0"
  Byte Unpack/1 -> Out17/1  "Wheel Speed Front Left"
  Selector7/1 -> Byte Unpack1/1  "Byte 0"
  Byte Unpack1/1 -> Out18/1  "Wheel Speed Front Right"
  CAN FD Unpack3/1 -> Selector11/1, Selector10/1, Selector9/1, Selector8/1  "BMS1"
  Selector8/1 -> Byte Unpack2/1  "Byte 0"
  Byte Unpack2/1 -> Out19/1  "BMS Current Sensor"
  Selector9/1 -> Byte Unpack3/1  "Byte 0"
  Byte Unpack3/1 -> Out20/1  "BMS Voltage"
  Selector10/1 -> Data Type Conversion18/1  "Byte 0"
  Data Type Conversion18/1 -> Out21/1  "BMS SOC"
  Selector11/1 -> Data Type Conversion19/1  "Byte 0"
  Data Type Conversion19/1 -> Out22/1  "BMS Temprature"
  CAN FD Unpack4/1 -> Selector15/1, Selector14/1, Selector13/1, Selector12/1  "BMS2"
  Selector12/1 -> Byte Unpack4/1  "Byte 0"
  Byte Unpack4/1 -> Terminator1/1  "DCL"
  Selector13/1 -> Byte Unpack5/1  "Byte 0"
  Byte Unpack5/1 -> Terminator2/1  "CCL"
  Selector14/1 -> Data Type Conversion20/1  "Byte 0"
  Data Type Conversion20/1 -> Out23/1  "BMS_Max_Cell_Temp"
  Selector15/1 -> Data Type Conversion21/1  "Byte 0"
  Data Type Conversion21/1 -> Out24/1  "BMS_Max_Cell_Temp"

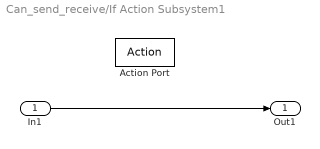
== system Can_send_receive/If Action Subsystem1 ==
  In1 : Inport
  Action Port : ActionPort  ActionPortLabel=case [ 138 ]:
  Out1 : Outport
  wires:
  In1/1 -> Out1/1

== system Can_send_receive/Subsystem ==
  Constant2 : Constant
  Out1 : Outport
  wires:
  Constant2/1 -> Out1/1

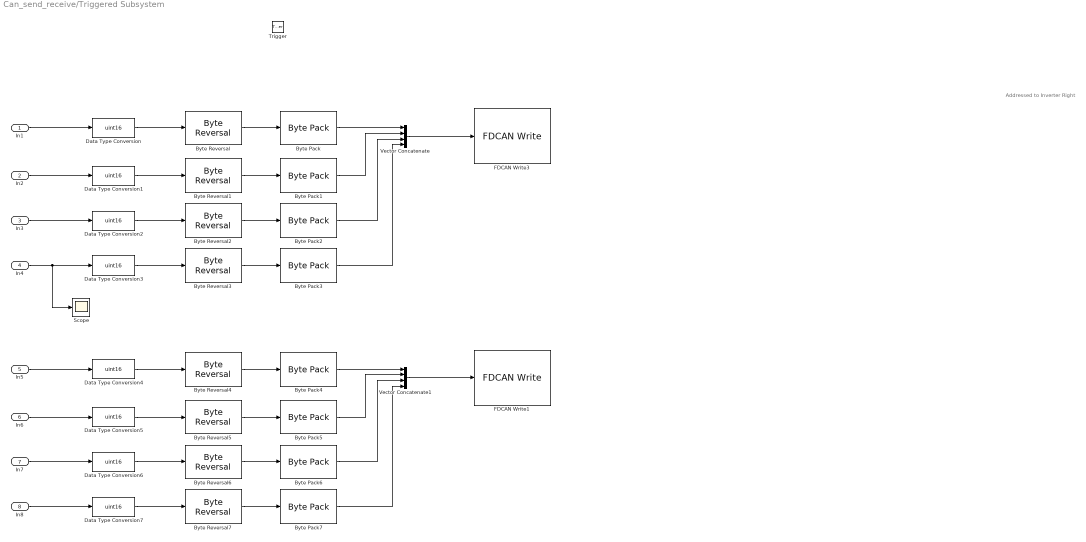
== system Can_send_receive/Triggered Subsystem ==
  note: Addressed to Inverter Right
  In1 : Inport
  In2 : Inport  Port=2
  In3 : Inport  Port=3
  In4 : Inport  Port=4
  In5 : Inport  Port=5
  In6 : Inport  Port=6
  In7 : Inport  Port=7
  In8 : Inport  Port=8
  Trigger : TriggerPort  TriggerType=function-call  VariantControl=(inherit)
  Byte Pack{,1..7} (8 alike) : stmutilitieslib/Byte Pack  datatypes={'uint16'}  byteAlign=1  blockPlatform=stm32f4discovery
  Byte Reversal{,1..7} (8 alike) : stmutilitieslib/Byte Reversal  numInp=1  blockPlatform=stm32f4discovery
  Data Type Conversion{,1..7} (8 alike) : DataTypeConversion  OutDataTypeStr=uint16  SaturateOnIntegerOverflow=off  RndMeth=Floor
  FDCAN Write1 : stm32blockslib/FDCAN Write  FDCANModule=FDCAN2  BlockMode=Transmit  OperationReadMode=Data  OperationWriteMode=Data  ReadSource=FIFO 0  BufferNumber=0  OutputTypeReadMode=Unpacked  DataFormatWriteMode=Raw data  CANFrameType=CAN  IdentifierTypeVia=Dialog  IdentifierType=Standard (11-bit identifier)  IdentifierVia=Dialog  Identifier=9  DataLengthVia=Dialog  DataLength=8  OutputIdType=off  IsBitRateSwitchingEnabled=off  TransmitRemoteFrame=off  OutputFrameType=off  OutputBRS=off  OutputRemoteFrame=off  OutputTxFifoLevel=off  OutputRxFifoLevel=off  OutputStatus=off  Timeout=1  SampleTime=-1
      settings: LibrarySourceBlock=stm32l5xxblockslib/FDCAN Write
  FDCAN Write3 : stm32blockslib/FDCAN Write  FDCANModule=FDCAN2  BlockMode=Transmit  OperationReadMode=Data  OperationWriteMode=Data  ReadSource=FIFO 0  BufferNumber=0  OutputTypeReadMode=Unpacked  DataFormatWriteMode=Raw data  CANFrameType=CAN  IdentifierTypeVia=Dialog  IdentifierType=Standard (11-bit identifier)  IdentifierVia=Dialog  Identifier=8  DataLengthVia=Dialog  DataLength=8  OutputIdType=off  IsBitRateSwitchingEnabled=off  TransmitRemoteFrame=off  OutputFrameType=off  OutputBRS=off  OutputRemoteFrame=off  OutputTxFifoLevel=off  OutputRxFifoLevel=off  OutputStatus=off  Timeout=1  SampleTime=-1
      settings: LibrarySourceBlock=stm32l5xxblockslib/FDCAN Write
  Scope : Scope
  Vector Concatenate : Concatenate  NumInputs=4
  Vector Concatenate1 : Concatenate  NumInputs=4
  wires:
  Byte Reversal/1 -> Byte Pack/1
  Byte Pack/1 -> Vector Concatenate/1
  Data Type Conversion/1 -> Byte Reversal/1
  In1/1 -> Data Type Conversion/1
  Byte Pack1/1 -> Vector Concatenate/2
  Byte Reversal1/1 -> Byte Pack1/1
  Data Type Conversion1/1 -> Byte Reversal1/1
  Byte Pack2/1 -> Vector Concatenate/3
  Byte Reversal2/1 -> Byte Pack2/1
  Data Type Conversion2/1 -> Byte Reversal2/1
  Byte Pack3/1 -> Vector Concatenate/4
  Byte Reversal3/1 -> Byte Pack3/1
  Data Type Conversion3/1 -> Byte Reversal3/1
  In2/1 -> Data Type Conversion1/1
  In3/1 -> Data Type Conversion2/1
  In4/1 -> Scope/1, Data Type Conversion3/1
  Vector Concatenate/1 -> FDCAN Write3/1
  Byte Pack6/1 -> Vector Concatenate1/3
  Byte Reversal7/1 -> Byte Pack7/1
  Vector Concatenate1/1 -> FDCAN Write1/1
  Byte Pack5/1 -> Vector Concatenate1/2
  Byte Pack7/1 -> Vector Concatenate1/4
  Byte Pack4/1 -> Vector Concatenate1/1
  Data Type Conversion7/1 -> Byte Reversal7/1
  Data Type Conversion4/1 -> Byte Reversal4/1
  Byte Reversal5/1 -> Byte Pack5/1
  Data Type Conversion5/1 -> Byte Reversal5/1
  Byte Reversal6/1 -> Byte Pack6/1
  Data Type Conversion6/1 -> Byte Reversal6/1
  Byte Reversal4/1 -> Byte Pack4/1
  In8/1 -> Data Type Conversion7/1
  In7/1 -> Data Type Conversion6/1
  In6/1 -> Data Type Conversion5/1
  In5/1 -> Data Type Conversion4/1

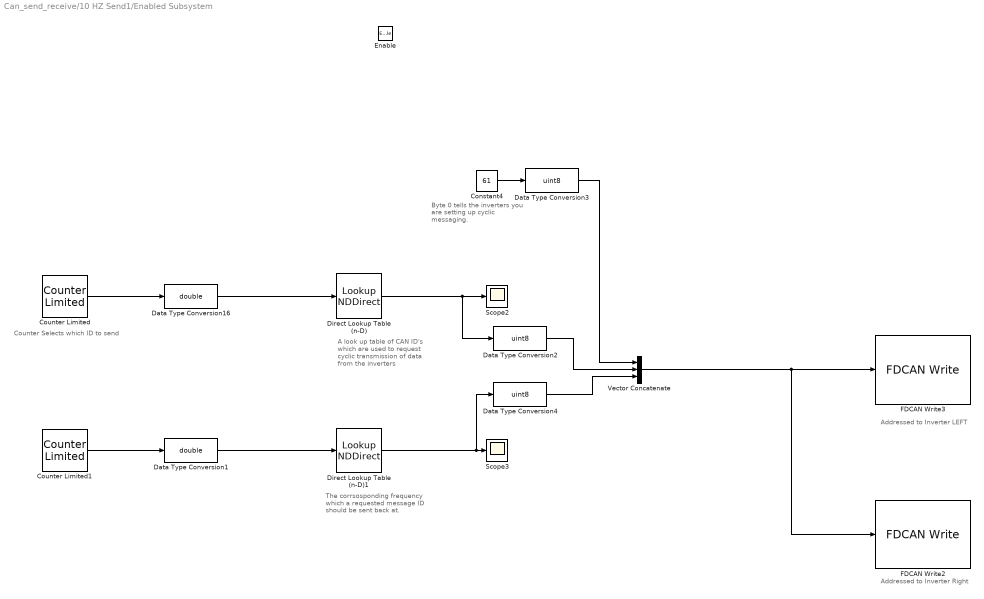
== system Can_send_receive/10 HZ Send1/Enabled Subsystem ==
  note: The corrsosponding frequency which a requested message ID should be sent back at.
  note: A look up table of CAN ID's which are used to request cyclic transmission of data from the inverters
  note: Byte 0 tells the inverters you are setting up cyclic messaging.
  note: Addressed to Inverter LEFT
  note: Counter Selects which ID to send
  note: Addressed to Inverter Right
  Enable : EnablePort
  Constant4 : Constant  Value=61
  Counter Limited : simulink/Sources/Counter Limited  uplimit=5  tsamp=-1
  Counter Limited1 : simulink/Sources/Counter Limited  uplimit=5  tsamp=-1
  Data Type Conversion1 : DataTypeConversion  OutDataTypeStr=double  SaturateOnIntegerOverflow=off  RndMeth=Floor
  Data Type Conversion16 : DataTypeConversion  OutDataTypeStr=double  SaturateOnIntegerOverflow=off  RndMeth=Floor
  Data Type Conversion2 : DataTypeConversion  OutDataTypeStr=uint8  SaturateOnIntegerOverflow=off  RndMeth=Floor
  Data Type Conversion3 : DataTypeConversion  OutDataTypeStr=uint8  SaturateOnIntegerOverflow=off  RndMeth=Floor
  Data Type Conversion4 : DataTypeConversion  OutDataTypeStr=uint8  SaturateOnIntegerOverflow=off  RndMeth=Floor
  Direct Lookup Table (n-D) : LookupNDDirect  NumberOfTableDimensions=1  Table=[235 74 168 73 95 138]
  Direct Lookup Table (n-D)1 : LookupNDDirect  NumberOfTableDimensions=1  Table=[235 74 168 73 95 138]
  FDCAN Write2 : stm32blockslib/FDCAN Write  FDCANModule=FDCAN2  BlockMode=Transmit  OperationReadMode=Data  OperationWriteMode=Data  ReadSource=FIFO 0  BufferNumber=0  OutputTypeReadMode=Unpacked  DataFormatWriteMode=Raw data  CANFrameType=CAN  IdentifierTypeVia=Dialog  IdentifierType=Standard (11-bit identifier)  IdentifierVia=Dialog  Identifier=529  DataLengthVia=Dialog  DataLength=3  OutputIdType=off  IsBitRateSwitchingEnabled=off  TransmitRemoteFrame=off  OutputFrameType=off  OutputBRS=off  OutputRemoteFrame=off  OutputTxFifoLevel=off  OutputRxFifoLevel=off  OutputStatus=off  Timeout=1  SampleTime=-1
      settings: LibrarySourceBlock=stm32l5xxblockslib/FDCAN Write
  FDCAN Write3 : stm32blockslib/FDCAN Write  FDCANModule=FDCAN2  BlockMode=Transmit  OperationReadMode=Data  OperationWriteMode=Data  ReadSource=FIFO 0  BufferNumber=0  OutputTypeReadMode=Unpacked  DataFormatWriteMode=Raw data  CANFrameType=CAN  IdentifierTypeVia=Dialog  IdentifierType=Standard (11-bit identifier)  IdentifierVia=Dialog  Identifier=528  DataLengthVia=Dialog  DataLength=3  OutputIdType=off  IsBitRateSwitchingEnabled=off  TransmitRemoteFrame=off  OutputFrameType=off  OutputBRS=off  OutputRemoteFrame=off  OutputTxFifoLevel=off  OutputRxFifoLevel=off  OutputStatus=off  Timeout=1  SampleTime=-1
      settings: LibrarySourceBlock=stm32l5xxblockslib/FDCAN Write
  Scope2 : Scope
  Scope3 : Scope
  Vector Concatenate : Concatenate  NumInputs=3
  wires:
  Direct Lookup Table (n-D)1/1 -> Data Type Conversion4/1, Scope3/1
  Data Type Conversion1/1 -> Direct Lookup Table (n-D)1/1
  Data Type Conversion16/1 -> Direct Lookup Table (n-D)/1
  Direct Lookup Table (n-D)/1 -> Data Type Conversion2/1, Scope2/1
  Counter Limited1/1 -> Data Type Conversion1/1
  Counter Limited/1 -> Data Type Conversion16/1
  Vector Concatenate/1 -> FDCAN Write2/1, FDCAN Write3/1
  Data Type Conversion3/1 -> Vector Concatenate/1
  Data Type Conversion4/1 -> Vector Concatenate/3
  Data Type Conversion2/1 -> Vector Concatenate/2
  Constant4/1 -> Data Type Conversion3/1

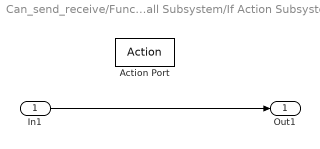
== system Can_send_receive/Function-Call Subsystem/If Action Subsystem1 ==
  In1 : Inport
  Action Port : ActionPort  ActionPortLabel=case [ 138 ]:
  Out1 : Outport
  wires:
  In1/1 -> Out1/1

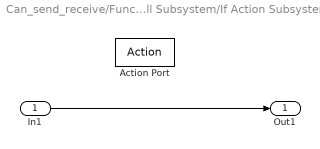
== system Can_send_receive/Function-Call Subsystem/If Action Subsystem10 ==
  In1 : Inport
  Action Port : ActionPort  ActionPortLabel=case [ 168 ]:
  Out1 : Outport
  wires:
  In1/1 -> Out1/1

== system Can_send_receive/Function-Call Subsystem/If Action Subsystem11 ==
  In1 : Inport
  Action Port : ActionPort  ActionPortLabel=case [ 74 ]:
  Out1 : Outport
  wires:
  In1/1 -> Out1/1

== system Can_send_receive/Function-Call Subsystem/If Action Subsystem12 ==
  In1 : Inport
  Action Port : ActionPort  ActionPortLabel=case [ 235 ]:
  Out1 : Outport
  wires:
  In1/1 -> Out1/1

== system Can_send_receive/Function-Call Subsystem/If Action Subsystem2 ==
  In1 : Inport
  Action Port : ActionPort  ActionPortLabel=case [ 95 ]:
  Out1 : Outport
  wires:
  In1/1 -> Out1/1

== system Can_send_receive/Function-Call Subsystem/If Action Subsystem3 ==
  In1 : Inport
  Action Port : ActionPort  ActionPortLabel=case [ 73 ]:
  Out1 : Outport
  wires:
  In1/1 -> Out1/1

== system Can_send_receive/Function-Call Subsystem/If Action Subsystem4 ==
  In1 : Inport
  Action Port : ActionPort  ActionPortLabel=case [ 168 ]:
  Out1 : Outport
  wires:
  In1/1 -> Out1/1

== system Can_send_receive/Function-Call Subsystem/If Action Subsystem5 ==
  In1 : Inport
  Action Port : ActionPort  ActionPortLabel=case [ 74 ]:
  Out1 : Outport
  wires:
  In1/1 -> Out1/1

== system Can_send_receive/Function-Call Subsystem/If Action Subsystem6 ==
  In1 : Inport
  Action Port : ActionPort  ActionPortLabel=case [ 235 ]:
  Out1 : Outport
  wires:
  In1/1 -> Out1/1

== system Can_send_receive/Function-Call Subsystem/If Action Subsystem7 ==
  In1 : Inport
  Action Port : ActionPort  ActionPortLabel=case [ 138 ]:
  Out1 : Outport
  wires:
  In1/1 -> Out1/1

== system Can_send_receive/Function-Call Subsystem/If Action Subsystem8 ==
  In1 : Inport
  Action Port : ActionPort  ActionPortLabel=case [ 95 ]:
  Out1 : Outport
  wires:
  In1/1 -> Out1/1

== system Can_send_receive/Function-Call Subsystem/If Action Subsystem9 ==
  In1 : Inport
  Action Port : ActionPort  ActionPortLabel=case [ 73 ]:
  Out1 : Outport
  wires:
  In1/1 -> Out1/1

== system Can_send_receive/Function-Call Subsystem1/Subsystem ==
  Constant2 : Constant
  Out1 : Outport
  wires:
  Constant2/1 -> Out1/1
